simulink model "tire_pacejka_model"  (R2025b)
settings: Solver=VariableStepAuto  StartTime=0.0  StopTime=10.0  RelTol=1e-3
settings Model: Creator=aborawake  LastModifiedBy=aborawake

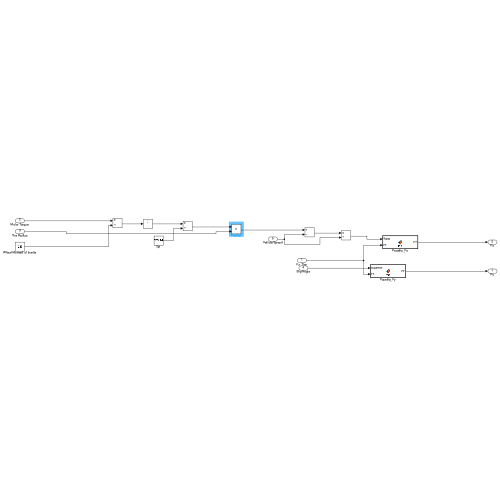
[thumbnail: Simulink's stored preview of the top-level diagram]
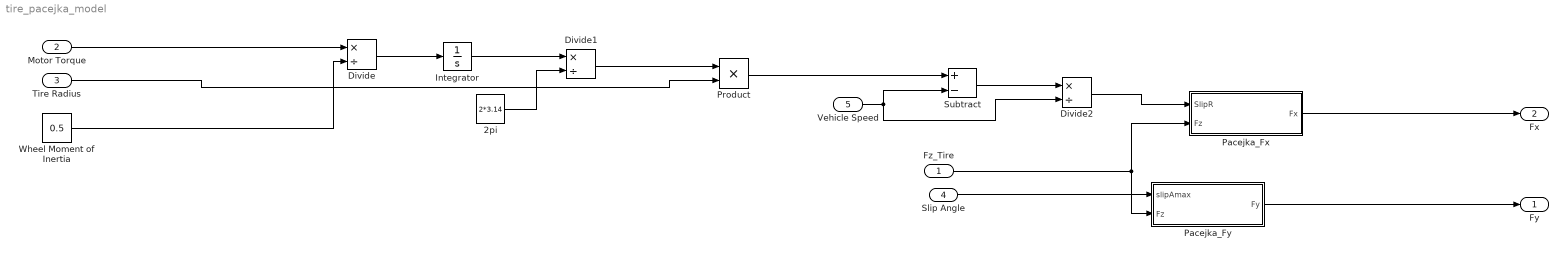
== system tire_pacejka_model ==
  Fz_Tire : Inport
  Motor Torque : Inport  Port=2
  Tire Radius : Inport  Port=3
  Slip Angle : Inport  Port=4
  Vehicle Speed : Inport  Port=5
  2pi : Constant  Value=2*3.14
  Divide : Product  Inputs=*/
  Divide1 : Product  Inputs=*/
  Divide2 : Product  Inputs=*/
  Integrator : Integrator
  Pacejka_Fx : MATLAB Function  TreatAsAtomicUnit=on
  Pacejka_Fy : MATLAB Function  TreatAsAtomicUnit=on
  Product : Product
  Subtract : Sum  Inputs=+-
  Wheel Moment of Inertia : Constant  Value=0.5
  Fy : Outport
  Fx : Outport  Port=2
  wires:
  Wheel Moment of Inertia/1 -> Divide/2
  Motor Torque/1 -> Divide/1
  Fz_Tire/1 -> Pacejka_Fx/2(Fz), Pacejka_Fy/2(Fz)
  Slip Angle/1 -> Pacejka_Fy/1(slipAmax)
  Divide/1 -> Integrator/1
  Integrator/1 -> Divide1/1
  Pacejka_Fy/1(Fy) -> Fy/1
  Pacejka_Fx/1(Fx) -> Fx/1
  2pi/1 -> Divide1/2
  Divide1/1 -> Product/1
  Tire Radius/1 -> Product/2
  Product/1 -> Subtract/1
  Vehicle Speed/1 -> Subtract/2, Divide2/2
  Subtract/1 -> Divide2/1
  Divide2/1 -> Pacejka_Fx/1(SlipR)

== matlab function tire_pacejka_model/Pacejka_Fx ==
  data: SlipR input; Fz input; Fx output
function Fx = fcn(SlipR, Fz)

    params = [ -15.75854662   1.43389415   3.343542286  0.91617855  ];

    B  = params(1);
    C  = params(2);
    D1 = params(3);
    D2 = params(4);
    
    D = (D1+D2/1000*Fz)*Fz;
    Fx = D*sin(C*atan(B*SlipRMax));

end

== matlab function tire_pacejka_model/Pacejka_Fy ==
  data: slipAmax input; Fy output; Fz input
function Fy = fcn(slipAmax, Fz)

    params = [   0.170613402  1.544452682  2.924301138  0.524592595 ];

    B  = params(1);
    C  = params(2);
    D1 = params(3);
    D2 = params(4);
    
    D = (D1+D2/1000*Fz)*Fz;
    Fy = -1*D*sin(C*atan(B*slipAmax));

end
